simulink model "simulation_doublePV_doubleBatt"  (R2020b)
settings: Solver=FixedStepAuto  StartTime=0.0  StopTime=sim_length  FixedStep=1  RelTol=1e-3
values from neighbouring files (symbols this model uses):
  air_delay = 0    [custom_exec_1.m]    (also in custom_exec_2.m = 30; parallel_exec.m; serial_exec.m)
  air_pulse = (air_time * 100)/period    (= 16.6666666667)    [custom_exec_1.m]    (also in custom_exec_2.m; parallel_exec.m; serial_exec.m = 5)
  battery_DCDC_current = importdata('battery_DCDC_current.mat')    [script.m]
  battery_DCDC_efficiency = importdata('battery_DCDC_efficiency.mat')    [script.m]
  G = [250; 500; 750; 1000]    [script.m]
  I = [I_250; I_500; I_750; I_1000]    [script.m]
  mc_delay = air_time + methane_time    (= 60)    [custom_exec_1.m]    (also in custom_exec_2.m; parallel_exec.m = 30; serial_exec.m = 78)
  mc_pulse = (mc_time*100)/period    (= 3.33333333333)    [custom_exec_1.m]    (also in custom_exec_2.m; parallel_exec.m; serial_exec.m = 1)
  methane_delay = air_time    (= 30)    [custom_exec_1.m]    (also in custom_exec_2.m = 0; parallel_exec.m = 0; serial_exec.m)
  methane_pulse = (methane_time * 100)/period    (= 16.6666666667)    [custom_exec_1.m]    (also in custom_exec_2.m; parallel_exec.m; serial_exec.m = 5)
  mic_delay = air_time    (= 30)    [custom_exec_1.m]    (also in custom_exec_2.m = 18; parallel_exec.m = 0; serial_exec.m = 66)
  mic_pulse = (mic_time * 100)/period    (= 6.66666666667)    [custom_exec_1.m]    (also in custom_exec_2.m; parallel_exec.m; serial_exec.m = 2)
  p1_R = -37.22    [script.m]
  p1_Voc = -143.6    [script.m]
  p2_R = 124.1    [script.m]
  p2_Voc = 504    [script.m]
  p3_R = -160.7    [script.m]
  p3_Voc = -692.3    [script.m]
  p4_R = 101.6    [script.m]
  p4_Voc = 471.7    [script.m]
  p5_R = -31.99    [script.m]
  p5_Voc = -165.2    [script.m]
  p6_R = 4.332    [script.m]
  p6_Voc = 29.02    [script.m]
  p7_R = 0.05868    [script.m]
  p7_Voc = 0.2082    [script.m]
  period = 180    [custom_exec_1.m]    (also in custom_exec_2.m; parallel_exec.m; serial_exec.m = 600)
  PV_DCDC_efficiency = importdata('PV_DCDC_efficiency.mat')    [script.m]
  PV_DCDC_voltage = importdata('PV_DCDC_voltage.mat')    [script.m]
  temp_delay = air_time+mic_time    (= 42)    [custom_exec_1.m]    (also in custom_exec_2.m = 12; parallel_exec.m = 0; serial_exec.m = 60)
  temp_pulse = (temp_time *100)/period    (= 3.33333333333)    [custom_exec_1.m]    (also in custom_exec_2.m; parallel_exec.m; serial_exec.m = 1)
  transmit_delay = mc_delay + mc_time    (= 66)    [custom_exec_1.m]    (also in custom_exec_2.m; parallel_exec.m = 36; serial_exec.m = 84)
  transmit_pulse = (transmit_time * 100)/period    (= 13.3333333333)    [custom_exec_1.m]    (also in custom_exec_2.m; parallel_exec.m; serial_exec.m = 4)
  V = [V_250; V_500; V_750; V_1000]    [script.m]
libraries: simulink x10
settings Model: Creator=sara  LastModifiedBy=Dario
settings DataIOCC: ReturnWorkspaceOutputs=off
settings DebuggingCC: ArithmeticOperatorsInVariantConditions=warning
settings SFSimCC: SimUseLocalCustomCode=off  CustomCodeUndefinedFunction=UseInterfaceOnly
settings RTWCC: RTWUseLocalCustomCode=off
settings CodeAppCC: StateflowObjectComments=on

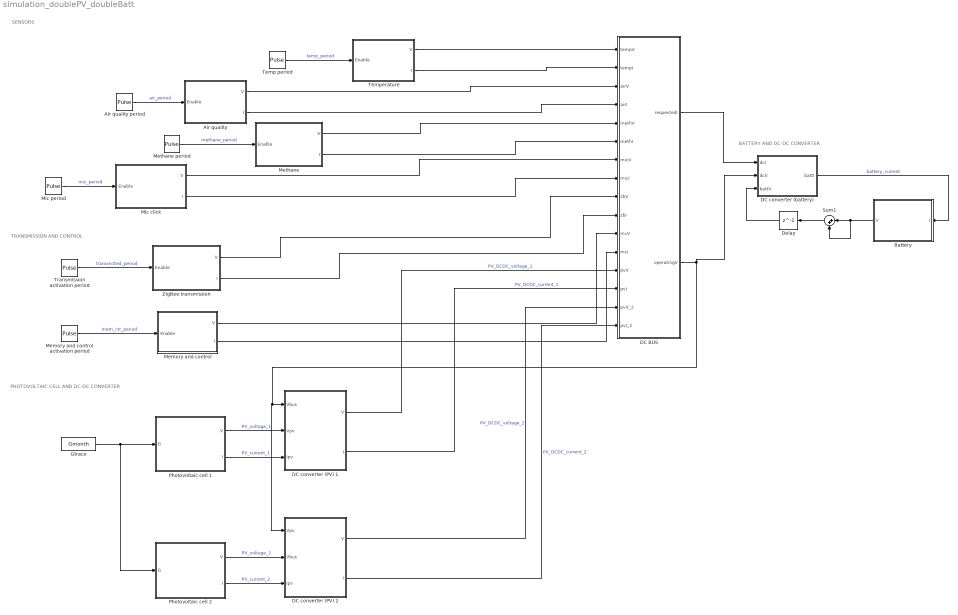
== system simulation_doublePV_doubleBatt ==
  note: TRANSMISSION AND CONTROL
  note: SENSORS
  note: PHOTOVOLTAIC CELL AND DC-DC CONVERTER
  note: BATTERY AND DC-DC CONVERTER
  Air quality : Subsystem
  Air quality period : DiscretePulseGenerator  PulseType=Time based  Period=period  PulseWidth=air_pulse  PhaseDelay=air_delay
  Battery : Subsystem
  DC BUS : Subsystem
  DC converter (PV) 1 : Subsystem
  DC converter (PV) 2 : Subsystem
  DC converter (battery) : Subsystem
  Delay : Delay  DelayLength=1  InitialCondition=0
  Gtrace : FromWorkspace  VariableName=Gmonth  OutputAfterFinalValue=Setting to zero
  Memory and control : Subsystem
  Memory and control activation period : DiscretePulseGenerator  PulseType=Time based  Period=period  PulseWidth=mc_pulse  PhaseDelay=mc_delay
  Methane : Subsystem
  Methane period : DiscretePulseGenerator  PulseType=Time based  Period=period  PulseWidth=methane_pulse  PhaseDelay=methane_delay
  Mic period : DiscretePulseGenerator  PulseType=Time based  Period=period  PulseWidth=mic_pulse  PhaseDelay=mic_delay
  Mic click : Subsystem
  Photovoltaic cell 1 : Subsystem
  Photovoltaic cell 2 : Subsystem
  Sum1 : Sum  Inputs=|++
  Temp period : DiscretePulseGenerator  PulseType=Time based  Period=period  PulseWidth=temp_pulse  PhaseDelay=temp_delay
  Temperature : Subsystem
  Transmission activation period : DiscretePulseGenerator  PulseType=Time based  Period=period  PulseWidth=transmit_pulse  PhaseDelay=transmit_delay
  ZigBee transmission : Subsystem
  wires:
  Mic click/2(I) -> DC BUS/8(micI)
  Mic click/1(V) -> DC BUS/7(micV)
  Mic period/1 -> Mic click/1(Enable)  "mic_period"
  Air quality period/1 -> Air quality/1(Enable)  "air_period"
  Air quality/1(V) -> DC BUS/3(airV)
  Air quality/2(I) -> DC BUS/4(airI)
  Methane/1(V) -> DC BUS/5(methV)
  Methane period/1 -> Methane/1(Enable)  "methane_period"
  Methane/2(I) -> DC BUS/6(methI)
  Temperature/1(V) -> DC BUS/1(tempV)
  Temp period/1 -> Temperature/1(Enable)  "temp_period"
  ZigBee transmission/1(V) -> DC BUS/9(zbV)
  Transmission activation period/1 -> ZigBee transmission/1(Enable)  "transmitted_period"
  Temperature/2(I) -> DC BUS/2(tempI)
  Memory and control/1(V) -> DC BUS/11(mcV)
  ZigBee transmission/2(I) -> DC BUS/10(zbI)
  Photovoltaic cell 1/1(V) -> DC converter (PV) 1/2(Vpv)  "PV_voltage_1"
  DC converter (battery)/1(battI) -> Battery/1(I)  "battery_current"
  DC BUS/1(requestedI) -> DC converter (battery)/1(dcI)
  Delay/1 -> DC converter (battery)/3(battV)
  Photovoltaic cell 1/2(I) -> DC converter (PV) 1/3(Ipv)  "PV_current_1"
  DC converter (PV) 1/2(I) -> DC BUS/14(pvI)  "PV_DCDC_current_1"
  DC converter (PV) 1/1(V) -> DC BUS/13(pvV)  "PV_DCDC_voltage_1"
  Memory and control/2(I) -> DC BUS/12(mcI)
  Memory and control activation period/1 -> Memory and control/1(Enable)  "mem_ctr_period"
  Gtrace/1 -> Photovoltaic cell 2/1(G), Photovoltaic cell 1/1(G)
  Photovoltaic cell 2/1(V) -> DC converter (PV) 2/2(Vbus)  "PV_voltage_2"
  Photovoltaic cell 2/2(I) -> DC converter (PV) 2/3(Ipv)  "PV_current_2"
  DC BUS/2(operatingV) -> DC converter (battery)/2(dcV), DC converter (PV) 2/1(Vpv), DC converter (PV) 1/1(Vbus)
  DC converter (PV) 2/1(V) -> DC BUS/15(pvV_2)  "PV_DCDC_voltage_2"
  DC converter (PV) 2/2(I) -> DC BUS/16(pvI_2)  "PV_DCDC_current_2"
  Sum1/1 -> Delay/1
  Battery/1(V) -> Sum1/2, Sum1/1

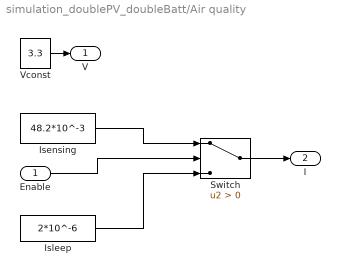
== system simulation_doublePV_doubleBatt/Air quality ==
  Enable : Inport
  Isensing : Constant  Value=48.2*10^-3
  Isleep : Constant  Value=2*10^-6
  Switch : Switch  Criteria=u2 > Threshold
  Vconst : Constant  Value=3.3
  V : Outport
  I : Outport  Port=2
  wires:
  Enable/1 -> Switch/2
  Isleep/1 -> Switch/3
  Vconst/1 -> V/1
  Isensing/1 -> Switch/1
  Switch/1 -> I/1

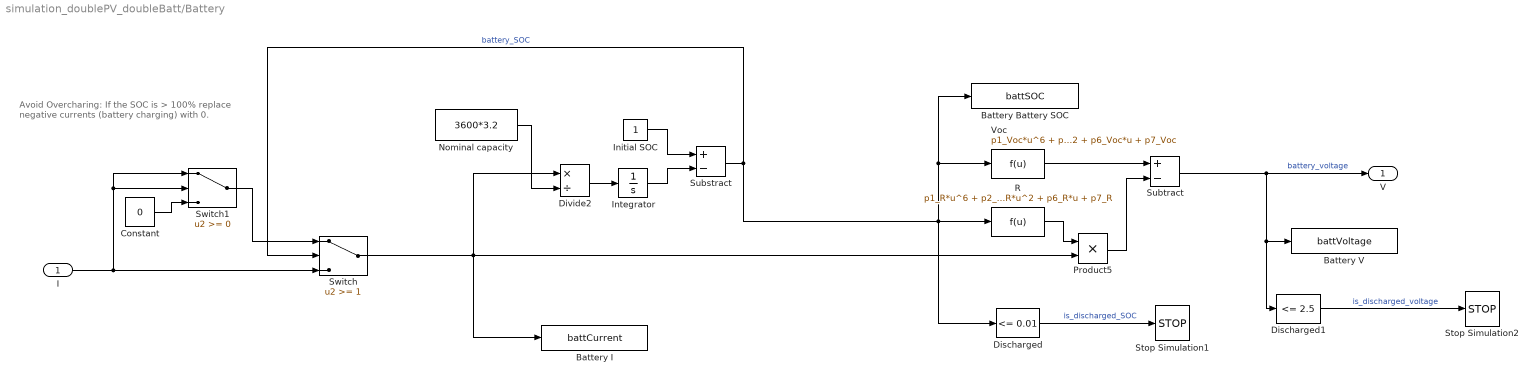
== system simulation_doublePV_doubleBatt/Battery ==
  note: Avoid Overcharing:
      | If the SOC is > 100% replace negative currents (battery charging) with 0.
  I : Inport
  Battery Battery SOC : ToWorkspace  VariableName=battSOC  SampleTime=-1
  Battery I : ToWorkspace  VariableName=battCurrent  SampleTime=-1
  Battery V : ToWorkspace  VariableName=battVoltage  SampleTime=-1
  Constant : Constant  Value=0
  Discharged : simulink/Logic and Bit Operations/Compare To Constant  relop=<=  const=0.01  OutDataTypeStr=boolean  ZeroCross=off
  Discharged1 : simulink/Logic and Bit Operations/Compare To Constant  relop=<=  const=2.5  OutDataTypeStr=boolean  ZeroCross=off
  Divide2 : Product  Inputs=*/
  Initial SOC : Constant
  Integrator : Integrator
  Nominal capacity : Constant  Value=3600*3.2
  Product5 : Product  RndMeth=Zero
  R : Fcn  Expr=p1_R*u^6 + p2_R*u^5 + p3_R*u^4 + p4_R*u^3 + p5_R*u^2 + p6_R*u + p7_R
  Stop Simulation1 : Stop
  Stop Simulation2 : Stop
  Substract : Sum  Inputs=+-
  Subtract : Sum  Inputs=+-
  Switch : Switch  Threshold=1
  Switch1 : Switch
  Voc : Fcn  Expr=p1_Voc*u^6 + p2_Voc*u^5 + p3_Voc*u^4 + p4_Voc*u^3 + p5_Voc*u^2 + p6_Voc*u + p7_Voc
  V : Outport
  wires:
  Integrator/1 -> Substract/2
  Nominal capacity/1 -> Divide2/2
  Divide2/1 -> Integrator/1
  Voc/1 -> Subtract/1
  Subtract/1 -> V/1, Battery V/1, Discharged1/1  "battery_voltage"
  I/1 -> Switch/3, Switch1/1, Switch1/2
  Product5/1 -> Subtract/2
  R/1 -> Product5/1
  Discharged/1 -> Stop Simulation1/1  "is_discharged_SOC"
  Initial SOC/1 -> Substract/1
  Discharged1/1 -> Stop Simulation2/1  "is_discharged_voltage"
  Substract/1 -> Voc/1, Battery Battery SOC/1, Discharged/1, R/1, Switch/2  "battery_SOC"
  Switch/1 -> Divide2/1, Product5/2, Battery I/1
  Switch1/1 -> Switch/1
  Constant/1 -> Switch1/3

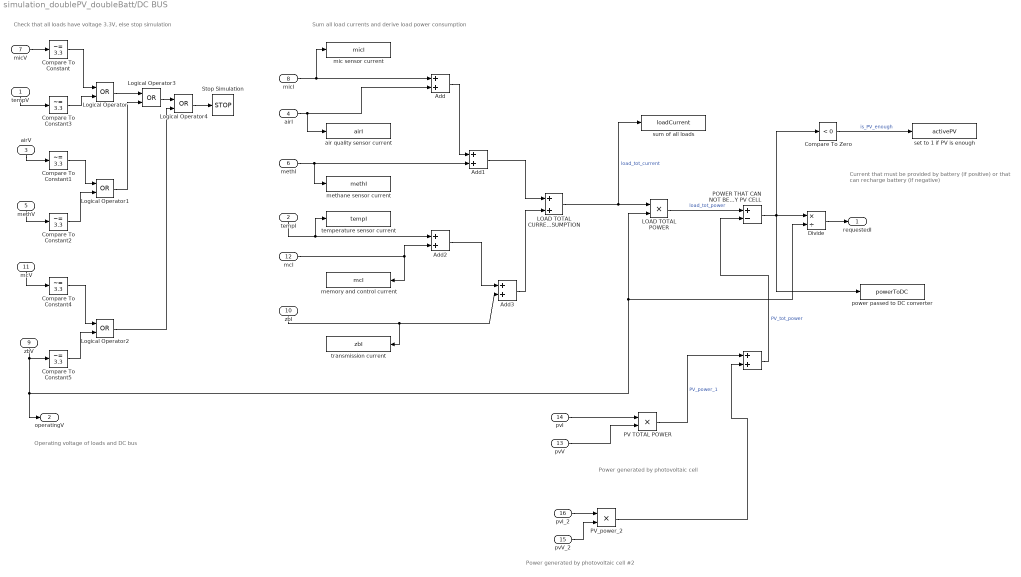
== system simulation_doublePV_doubleBatt/DC BUS ==
  note: Check that all loads have voltage 3.3V, else stop simulation
  note: Sum all load currents and derive load power consumption
  note: Power generated by photovoltaic cell
  note: Current that must be provided by battery (if positive) or that can recharge battery (if negative)
  note: Operating voltage of loads and DC bus
  note: Power generated by photovoltaic cell #2
  tempV : Inport
  tempI : Inport  Port=2
  airV : Inport  Port=3
  airI : Inport  Port=4
  methV : Inport  Port=5
  methI : Inport  Port=6
  micV : Inport  Port=7
  micI : Inport  Port=8
  zbV : Inport  Port=9
  zbI : Inport  Port=10
  mcV : Inport  Port=11
  mcI : Inport  Port=12
  pvV : Inport  Port=13
  pvI : Inport  Port=14
  pvV_2 : Inport  Port=15
  pvI_2 : Inport  Port=16
  "  " : Sum
  Add{,1..3} (4 alike) : Sum
  Compare To Constant{,1..5} (6 alike) : simulink/Logic and Bit Operations/Compare To Constant  relop=~=  const=3.3  OutDataTypeStr=boolean
  Compare To Zero : simulink/Logic and Bit Operations/Compare To Zero  relop=<  OutDataTypeStr=boolean
  Divide : Product  Inputs=*/
  LOAD TOTAL CURRENT CONSUMPTION : Sum
  LOAD TOTAL POWER : Product
  Logical Operator{,1..4} (5 alike) : Logic  Operator=OR  AllPortsSameDT=off  OutDataTypeStr=boolean
  POWER THAT CAN NOT BE PROVIDED BY PV CELL : Sum  Inputs=+-
  PV TOTAL POWER : Product
  PV_power_2 : Product
  Stop Simulation : Stop
  air quality sensor current : ToWorkspace  VariableName=airI  SampleTime=-1
  memory and control current : ToWorkspace  VariableName=mcI  SampleTime=-1
  methane sensor current : ToWorkspace  VariableName=methI  SampleTime=-1
  mic sensor current : ToWorkspace  VariableName=micI  SampleTime=-1
  power passed to DC converter : ToWorkspace  VariableName=powerToDC  SampleTime=-1
  set to 1 if PV is enough : ToWorkspace  VariableName=activePV  SampleTime=-1
  sum of all loads : ToWorkspace  VariableName=loadCurrent  SampleTime=-1
  temperature sensor current : ToWorkspace  VariableName=tempI  SampleTime=-1
  transmission current : ToWorkspace  VariableName=zbI  SampleTime=-1
  requestedI : Outport
  operatingV : Outport  Port=2
  wires:
  airV/1 -> Compare To Constant1/1
  Add/1 -> Add1/1
  zbV/1 -> operatingV/1, Divide/2, LOAD TOTAL POWER/2, Compare To Constant5/1
  methI/1 -> methane sensor current/1, Add1/2
  methV/1 -> Compare To Constant2/1
  micV/1 -> Compare To Constant/1
  micI/1 -> mic sensor current/1, Add/1
  mcV/1 -> Compare To Constant4/1
  Add3/1 -> LOAD TOTAL CURRENT CONSUMPTION/2
  airI/1 -> air quality sensor current/1, Add/2
  Add1/1 -> LOAD TOTAL CURRENT CONSUMPTION/1
  tempV/1 -> Compare To Constant3/1
  Compare To Constant/1 -> Logical Operator/1
  Compare To Constant3/1 -> Logical Operator/2
  Compare To Constant1/1 -> Logical Operator1/1
  Compare To Constant2/1 -> Logical Operator1/2
  Compare To Constant4/1 -> Logical Operator2/1
  Compare To Constant5/1 -> Logical Operator2/2
  Logical Operator/1 -> Logical Operator3/1
  Logical Operator1/1 -> Logical Operator3/2
  Logical Operator3/1 -> Logical Operator4/1
  Logical Operator2/1 -> Logical Operator4/2
  Logical Operator4/1 -> Stop Simulation/1
  mcI/1 -> Add2/2, memory and control current/1
  tempI/1 -> temperature sensor current/1, Add2/1
  Add2/1 -> Add3/1
  zbI/1 -> transmission current/1, Add3/2
  pvI/1 -> PV TOTAL POWER/1
  pvV/1 -> PV TOTAL POWER/2
  LOAD TOTAL CURRENT CONSUMPTION/1 -> sum of all loads/1, LOAD TOTAL POWER/1  "load_tot_current"
  LOAD TOTAL POWER/1 -> POWER THAT CAN NOT BE PROVIDED BY PV CELL/1  "load_tot_power"
  "  "/1 -> POWER THAT CAN NOT BE PROVIDED BY PV CELL/2  "PV_tot_power"
  POWER THAT CAN NOT BE PROVIDED BY PV CELL/1 -> power passed to DC converter/1, Compare To Zero/1, Divide/1
  Divide/1 -> requestedI/1
  Compare To Zero/1 -> set to 1 if PV is enough/1  "is_PV_enough"
  pvV_2/1 -> PV_power_2/2
  PV_power_2/1 -> "  "/2
  pvI_2/1 -> PV_power_2/1
  PV TOTAL POWER/1 -> "  "/1  "PV_power_1"

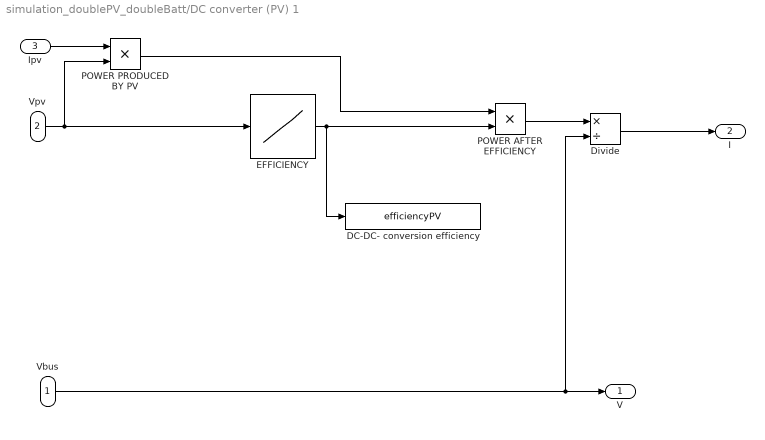
== system simulation_doublePV_doubleBatt/DC converter (PV) 1 ==
  Vbus : Inport
  Vpv : Inport  Port=2
  Ipv : Inport  Port=3
  DC-DC- conversion efficiency : ToWorkspace  VariableName=efficiencyPV  SampleTime=-1
  Divide : Product  Inputs=*/
  EFFICIENCY : Lookup_n-D  NumberOfTableDimensions=1  BreakpointsForDimension1=PV_DCDC_voltage  Table=PV_DCDC_efficiency  InternalRulePriority=Speed  RndMeth=Simplest  InputSameDT=on
  POWER PRODUCED BY PV : Product
  "POWER AFTER EFFICIENCY " : Product
  V : Outport
  I : Outport  Port=2
  wires:
  "POWER AFTER EFFICIENCY "/1 -> Divide/1
  Vbus/1 -> Divide/2, V/1
  POWER PRODUCED BY PV/1 -> "POWER AFTER EFFICIENCY "/1
  Divide/1 -> I/1
  EFFICIENCY/1 -> DC-DC- conversion efficiency/1, "POWER AFTER EFFICIENCY "/2
  Ipv/1 -> POWER PRODUCED BY PV/1
  Vpv/1 -> POWER PRODUCED BY PV/2, EFFICIENCY/1

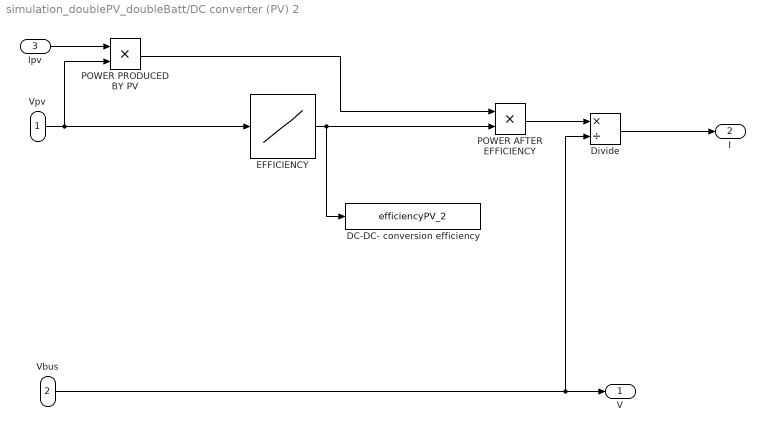
== system simulation_doublePV_doubleBatt/DC converter (PV) 2 ==
  Vpv : Inport
  Vbus : Inport  Port=2
  Ipv : Inport  Port=3
  DC-DC- conversion efficiency : ToWorkspace  VariableName=efficiencyPV_2  SampleTime=-1
  Divide : Product  Inputs=*/
  EFFICIENCY : Lookup_n-D  NumberOfTableDimensions=1  BreakpointsForDimension1=PV_DCDC_voltage  Table=PV_DCDC_efficiency  InternalRulePriority=Speed  RndMeth=Simplest  InputSameDT=on
  POWER PRODUCED BY PV : Product
  "POWER AFTER EFFICIENCY " : Product
  V : Outport
  I : Outport  Port=2
  wires:
  "POWER AFTER EFFICIENCY "/1 -> Divide/1
  Vbus/1 -> Divide/2, V/1
  POWER PRODUCED BY PV/1 -> "POWER AFTER EFFICIENCY "/1
  Divide/1 -> I/1
  EFFICIENCY/1 -> DC-DC- conversion efficiency/1, "POWER AFTER EFFICIENCY "/2
  Ipv/1 -> POWER PRODUCED BY PV/1
  Vpv/1 -> POWER PRODUCED BY PV/2, EFFICIENCY/1

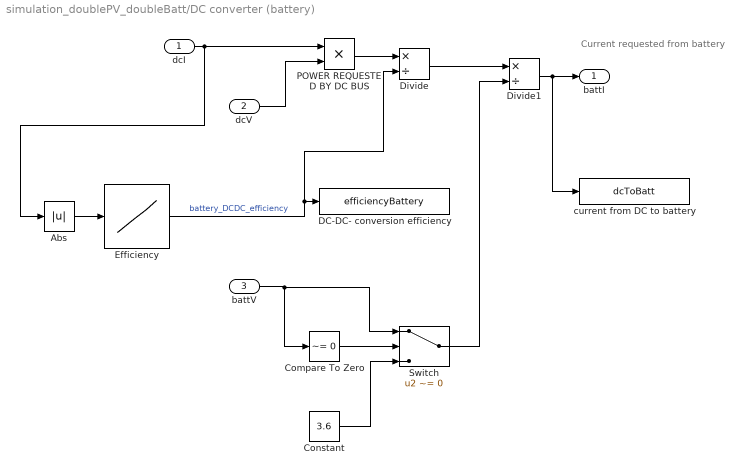
== system simulation_doublePV_doubleBatt/DC converter (battery) ==
  note: Current requested from battery
  dcI : Inport
  dcV : Inport  Port=2
  battV : Inport  Port=3
  Abs : Abs
  Compare To Zero : simulink/Logic and Bit Operations/Compare To Zero  relop=~=  OutDataTypeStr=boolean
  Constant : Constant  Value=3.6
  DC-DC- conversion efficiency : ToWorkspace  VariableName=efficiencyBattery  SampleTime=-1
  Divide : Product  Inputs=*/
  Divide1 : Product  Inputs=*/
  Efficiency : Lookup_n-D  NumberOfTableDimensions=1  BreakpointsForDimension1=battery_DCDC_current  Table=battery_DCDC_efficiency  InternalRulePriority=Speed  RndMeth=Simplest  InputSameDT=on
  POWER REQUESTED BY DC BUS : Product
  Switch : Switch  Criteria=u2 ~= 0
  current from DC to battery : ToWorkspace  VariableName=dcToBatt  SampleTime=-1
  battI : Outport
  wires:
  dcV/1 -> POWER REQUESTED BY DC BUS/2
  POWER REQUESTED BY DC BUS/1 -> Divide/1
  Divide/1 -> Divide1/1
  Divide1/1 -> current from DC to battery/1, battI/1
  dcI/1 -> Abs/1, POWER REQUESTED BY DC BUS/1
  battV/1 -> Switch/1, Compare To Zero/1
  Compare To Zero/1 -> Switch/2
  Constant/1 -> Switch/3
  Switch/1 -> Divide1/2
  Efficiency/1 -> Divide/2, DC-DC- conversion efficiency/1  "battery_DCDC_efficiency"
  Abs/1 -> Efficiency/1

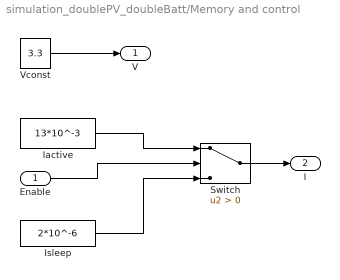
== system simulation_doublePV_doubleBatt/Memory and control ==
  Enable : Inport
  Iactive : Constant  Value=13*10^-3
  Isleep : Constant  Value=2*10^-6
  Switch : Switch  Criteria=u2 > Threshold
  Vconst : Constant  Value=3.3
  V : Outport
  I : Outport  Port=2
  wires:
  Vconst/1 -> V/1
  Iactive/1 -> Switch/1
  Switch/1 -> I/1
  Isleep/1 -> Switch/3
  Enable/1 -> Switch/2

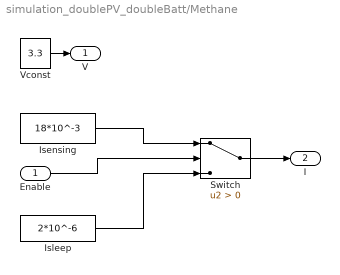
== system simulation_doublePV_doubleBatt/Methane ==
  Enable : Inport
  Isensing : Constant  Value=18*10^-3
  Isleep : Constant  Value=2*10^-6
  Switch : Switch  Criteria=u2 > Threshold
  Vconst : Constant  Value=3.3
  V : Outport
  I : Outport  Port=2
  wires:
  Enable/1 -> Switch/2
  Isleep/1 -> Switch/3
  Vconst/1 -> V/1
  Isensing/1 -> Switch/1
  Switch/1 -> I/1

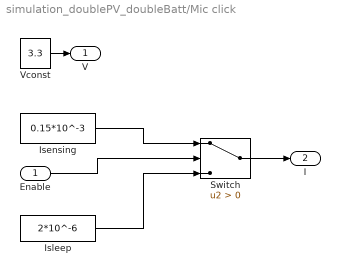
== system simulation_doublePV_doubleBatt/Mic click ==
  Enable : Inport
  Isensing : Constant  Value=0.15*10^-3
  Isleep : Constant  Value=2*10^-6
  Switch : Switch  Criteria=u2 > Threshold
  Vconst : Constant  Value=3.3
  V : Outport
  I : Outport  Port=2
  wires:
  Enable/1 -> Switch/2
  Isleep/1 -> Switch/3
  Vconst/1 -> V/1
  Isensing/1 -> Switch/1
  Switch/1 -> I/1

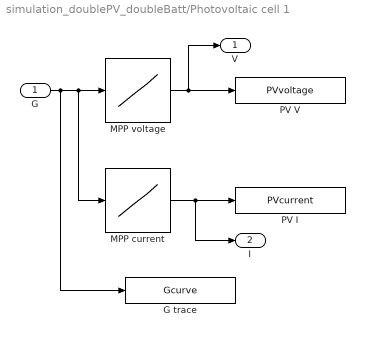
== system simulation_doublePV_doubleBatt/Photovoltaic cell 1 ==
  G : Inport
  G trace : ToWorkspace  VariableName=Gcurve  SampleTime=-1
  MPP current : Lookup_n-D  NumberOfTableDimensions=1  BreakpointsForDimension1=G  Table=I  InternalRulePriority=Speed  RndMeth=Simplest  InputSameDT=on
  MPP voltage : Lookup_n-D  NumberOfTableDimensions=1  BreakpointsForDimension1=G  Table=V  InternalRulePriority=Speed  RndMeth=Simplest  InputSameDT=on
  PV I : ToWorkspace  VariableName=PVcurrent  SampleTime=-1
  PV V : ToWorkspace  VariableName=PVvoltage  SampleTime=-1
  V : Outport
  I : Outport  Port=2
  wires:
  MPP voltage/1 -> PV V/1, V/1
  MPP current/1 -> PV I/1, I/1
  G/1 -> G trace/1, MPP current/1, MPP voltage/1

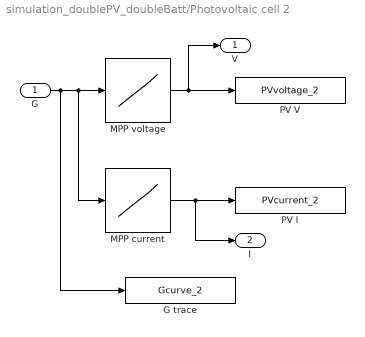
== system simulation_doublePV_doubleBatt/Photovoltaic cell 2 ==
  G : Inport
  G trace : ToWorkspace  VariableName=Gcurve_2  SampleTime=-1
  MPP current : Lookup_n-D  NumberOfTableDimensions=1  BreakpointsForDimension1=G  Table=I  InternalRulePriority=Speed  RndMeth=Simplest  InputSameDT=on
  MPP voltage : Lookup_n-D  NumberOfTableDimensions=1  BreakpointsForDimension1=G  Table=V  InternalRulePriority=Speed  RndMeth=Simplest  InputSameDT=on
  PV I : ToWorkspace  VariableName=PVcurrent_2  SampleTime=-1
  PV V : ToWorkspace  VariableName=PVvoltage_2  SampleTime=-1
  V : Outport
  I : Outport  Port=2
  wires:
  MPP voltage/1 -> PV V/1, V/1
  MPP current/1 -> PV I/1, I/1
  G/1 -> G trace/1, MPP current/1, MPP voltage/1

== system simulation_doublePV_doubleBatt/Temperature ==
  Enable : Inport
  Isensing : Constant  Value=0.3*10^-3
  Isleep : Constant  Value=2*10^-6
  Switch : Switch  Criteria=u2 > Threshold
  Vconst : Constant  Value=3.3
  V : Outport
  I : Outport  Port=2
  wires:
  Enable/1 -> Switch/2
  Isleep/1 -> Switch/3
  Vconst/1 -> V/1
  Isensing/1 -> Switch/1
  Switch/1 -> I/1

== system simulation_doublePV_doubleBatt/ZigBee transmission ==
  Enable : Inport
  Iidle : Constant  Value=1*10^-6
  Itransmitting : Constant  Value=0.1*10^-3
  Switch : Switch  Criteria=u2 > Threshold
  Vconst : Constant  Value=3.3
  V : Outport
  I : Outport  Port=2
  wires:
  Enable/1 -> Switch/2
  Iidle/1 -> Switch/3
  Vconst/1 -> V/1
  Itransmitting/1 -> Switch/1
  Switch/1 -> I/1
